simulink model "RcvyRStateCtrl"  (R2018b)
settings: Solver=FixedStepDiscrete  StartTime=0.0  StopTime=10.0  FixedStep=0.01  RelTol=1e-3
libraries: StateCtrlLib x1
settings Model: Creator=sn2xws  LastModifiedBy=sn2xws
settings DataIOCC: SaveFormat=StructureWithTime
settings OptimizationCC: DefaultParameterBehavior=Inlined  EnhancedBackFolding=on  PassReuseOutputArgsAs=Individual arguments  ZeroExternalMemoryAtStartup=off  ZeroInternalMemoryAtStartup=off  OptimizeBlockOrder=speed  DifferentSizesBufferReuse=on  OptimizationCustomize=off
settings DebuggingCC: ParameterTunabilityLossMsg=error
settings ModelReferenceCC: ModelReferenceNumInstancesAllowed=Single
settings SFSimCC: MATLABDynamicMemAlloc=off
settings RTWCC: SystemTargetFile=autosar.tlc  GenCodeOnly=on  TemplateMakefile=ert_default_tmf  Description=AUTOSAR  GenerateReport=on  IncludeHyperlinkInReport=on  LaunchReport=on  GenerateTraceInfo=on  GenerateTraceReport=on  GenerateTraceReportSl=on  GenerateTraceReportSf=on  GenerateTraceReportEml=on
settings CodeAppCC: ForceParamTrailComments=on  IgnoreCustomStorageClasses=off  OperatorAnnotations=on  SimulinkDataObjDesc=on  SFDataObjDesc=on  InsertBlockDesc=on
settings STFCustomTargetCC: TargetLangStandard=C99 (ISO)  MultiwordLength=256  ParMdlRefBuildCompliant=on  CompOptLevelCompliant=on  IncludeMdlTerminateFcn=off  CombineOutputUpdateFcns=on  SuppressErrorStatus=on  ERTCustomFileBanners=on  SupportNonFinite=off  SupportComplex=off  SupportContinuousTime=off  SupportNonInlinedSFcns=off  RemoveResetFunc=on  MATLABClassNameForMDSCustomization=Simulink.SoftwareTarget.ERTCustomization  AutosarCompliant=on  UseToolchainInfoCompliant=on  LookupTableObjectStructAxisOrder=2,1,3,4,...  LUTObjectStructOrderEvenSpacing=Size,Table,Breakpoints  SystemTargetFile=autosar.tlc
settings ERTTargetCC: TargetLangStandard=C99 (ISO)  ConcurrentExecutionCompliant=off  IncludeMdlTerminateFcn=off  SuppressErrorStatus=on  SupportNonFinite=off  SupportComplex=off  ModelStepFunctionPrototypeControlCompliant=off  CPPClassGenCompliant=off  AutosarCompliant=on  LookupTableObjectStructAxisOrder=2,1,3,4,...  LUTObjectStructOrderEvenSpacing=Size,Table,Breakpoints  InlinedParameterPlacement=NonHierarchical  ERTCustomFileTemplate=example_file_process.tlc

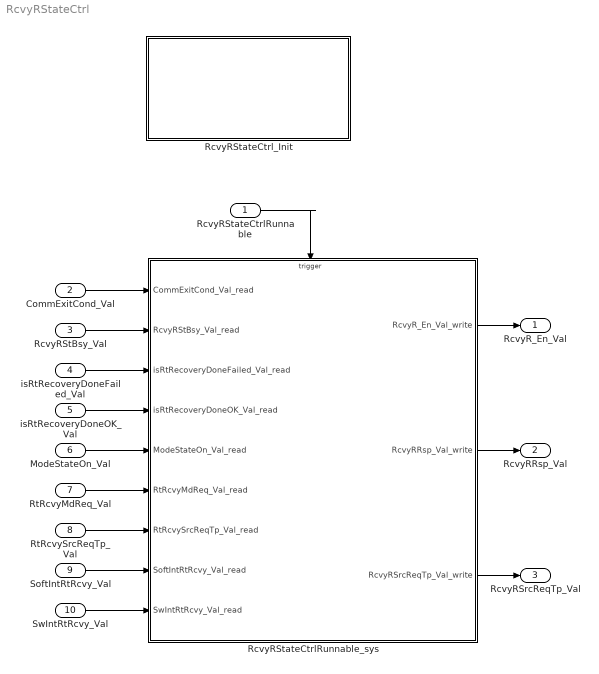
== system RcvyRStateCtrl ==
  RcvyRStateCtrlRunnable : Inport  SampleTime=0.01  OutputFunctionCall=on
  CommExitCond_Val : Inport  Port=2  OutDataTypeStr=boolean  PortDimensions=1
  RcvyRStBsy_Val : Inport  Port=3  OutDataTypeStr=boolean  PortDimensions=1
  isRtRecoveryDoneFailed_Val : Inport  Port=4  OutDataTypeStr=boolean  PortDimensions=1
  isRtRecoveryDoneOK_Val : Inport  Port=5  OutDataTypeStr=boolean  PortDimensions=1
  ModeStateOn_Val : Inport  Port=6  OutDataTypeStr=boolean  PortDimensions=1
  RtRcvyMdReq_Val : Inport  Port=7  OutDataTypeStr=boolean  PortDimensions=1
  RtRcvySrcReqTp_Val : Inport  Port=8  OutDataTypeStr=Enum: SrcReqTp1  PortDimensions=1
  SoftIntRtRcvy_Val : Inport  Port=9  OutDataTypeStr=IntEnable  PortDimensions=1
  SwIntRtRcvy_Val : Inport  Port=10  OutDataTypeStr=IntEnable  PortDimensions=1
  RcvyRStateCtrlRunnable_sys : Subsystem
  RcvyRStateCtrl_Init : Subsystem
  RcvyR_En_Val : Outport  OutDataTypeStr=boolean  PortDimensions=1
  RcvyRRsp_Val : Outport  Port=2  OutDataTypeStr=Enum: MdRspLocal1  PortDimensions=1
  RcvyRSrcReqTp_Val : Outport  Port=3  OutDataTypeStr=Enum: SrcReqTp1  PortDimensions=1
  wires:
  CommExitCond_Val/1 -> RcvyRStateCtrlRunnable_sys/1(CommExitCond_Val_read)
  RcvyRStBsy_Val/1 -> RcvyRStateCtrlRunnable_sys/2(RcvyRStBsy_Val_read)
  isRtRecoveryDoneFailed_Val/1 -> RcvyRStateCtrlRunnable_sys/3(isRtRecoveryDoneFailed_Val_read)
  isRtRecoveryDoneOK_Val/1 -> RcvyRStateCtrlRunnable_sys/4(isRtRecoveryDoneOK_Val_read)
  ModeStateOn_Val/1 -> RcvyRStateCtrlRunnable_sys/5(ModeStateOn_Val_read)
  RtRcvyMdReq_Val/1 -> RcvyRStateCtrlRunnable_sys/6(RtRcvyMdReq_Val_read)
  RtRcvySrcReqTp_Val/1 -> RcvyRStateCtrlRunnable_sys/7(RtRcvySrcReqTp_Val_read)
  SoftIntRtRcvy_Val/1 -> RcvyRStateCtrlRunnable_sys/8(SoftIntRtRcvy_Val_read)
  SwIntRtRcvy_Val/1 -> RcvyRStateCtrlRunnable_sys/9(SwIntRtRcvy_Val_read)
  RcvyRStateCtrlRunnable_sys/1(RcvyR_En_Val_write) -> RcvyR_En_Val/1
  RcvyRStateCtrlRunnable_sys/2(RcvyRRsp_Val_write) -> RcvyRRsp_Val/1
  RcvyRStateCtrlRunnable_sys/3(RcvyRSrcReqTp_Val_write) -> RcvyRSrcReqTp_Val/1
  RcvyRStateCtrlRunnable/1 -> RcvyRStateCtrlRunnable_sys/Trigger

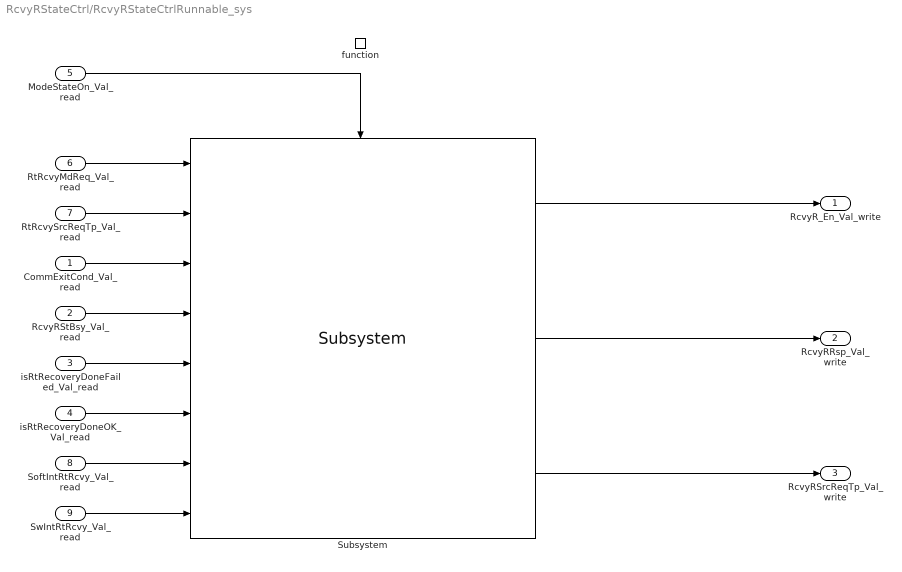
== system RcvyRStateCtrl/RcvyRStateCtrlRunnable_sys ==
  CommExitCond_Val_read : Inport
  RcvyRStBsy_Val_read : Inport  Port=2
  isRtRecoveryDoneFailed_Val_read : Inport  Port=3
  isRtRecoveryDoneOK_Val_read : Inport  Port=4
  ModeStateOn_Val_read : Inport  Port=5
  RtRcvyMdReq_Val_read : Inport  Port=6
  RtRcvySrcReqTp_Val_read : Inport  Port=7
  SoftIntRtRcvy_Val_read : Inport  Port=8  OutDataTypeStr=IntEnable
  SwIntRtRcvy_Val_read : Inport  Port=9  OutDataTypeStr=IntEnable
  function : TriggerPort  TriggerType=function-call  VariantControl=(inherit)  SampleTimeType=periodic  SampleTime=-1
  Subsystem : StateCtrlLib/Subsystem  SystemSampleTime=-1
  RcvyR_En_Val_write : Outport
      settings: EnsureOutportIsVirtual=on
  RcvyRRsp_Val_write : Outport  Port=2
      settings: EnsureOutportIsVirtual=on
  RcvyRSrcReqTp_Val_write : Outport  Port=3
      settings: EnsureOutportIsVirtual=on
  wires:
  Subsystem/2 -> RcvyRRsp_Val_write/1
  Subsystem/1 -> RcvyR_En_Val_write/1
  Subsystem/3 -> RcvyRSrcReqTp_Val_write/1
  ModeStateOn_Val_read/1 -> Subsystem/Enable
  RtRcvyMdReq_Val_read/1 -> Subsystem/1
  RtRcvySrcReqTp_Val_read/1 -> Subsystem/2
  CommExitCond_Val_read/1 -> Subsystem/3
  SoftIntRtRcvy_Val_read/1 -> Subsystem/7
  RcvyRStBsy_Val_read/1 -> Subsystem/4
  SwIntRtRcvy_Val_read/1 -> Subsystem/8
  isRtRecoveryDoneFailed_Val_read/1 -> Subsystem/5
  isRtRecoveryDoneOK_Val_read/1 -> Subsystem/6

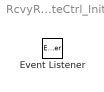
== system RcvyRStateCtrl/RcvyRStateCtrl_Init ==
  Event Listener : EventListener  EventName=reset
